simulink model "Model_R2021b"  (R2022b)
settings: Solver=VariableStepAuto  StartTime=0.0  StopTime=10  FixedStep=1e-5  RelTol=1e-3
InitFcn:
  | ModelParameters
values from neighbouring files (symbols this model uses):
  K = lqr(sys, Q, R)    [ModelParameters.m]
  U_ss = [m*g; 0; 0; 0]    [ModelParameters.m]
  X_init = [1.,1.,1.,  0,0,0,  0,0,psi_0, 0,0,0]    [ModelParameters.m]
  X_ref = [0,0,0, 0,0,0, 0,0,psi_t, 0,0,0]    [ModelParameters.m]
settings Model: Creator=samuel  LastModifiedBy=sebas
settings SolverCC: ZeroCrossControl=DisableAll  AlgebraicLoopSolver=TrustRegion
settings DebuggingCC: UnconnectedInputMsg=warning  UnconnectedOutputMsg=warning  UnconnectedLineMsg=warning  UnderSpecifiedDimensionMsg=warning  ArithmeticOperatorsInVariantConditions=warning
settings ModelReferenceCC: EnableRefExpFcnMdlSchedulingChecks=on
settings SFSimCC: CustomCodeUndefinedFunction=UseInterfaceOnly
settings RTWCC: DLArmComputeVersion=19.05

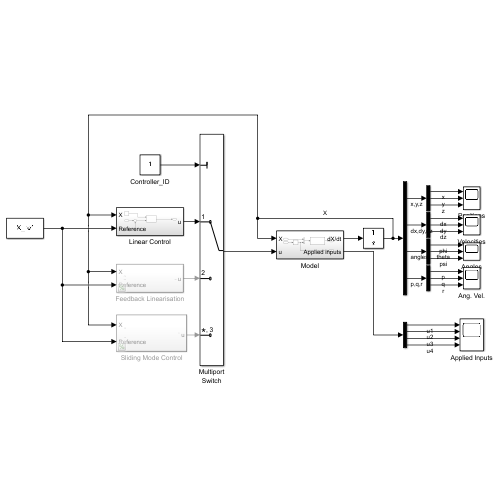
[thumbnail: Simulink's stored preview of the top-level diagram]
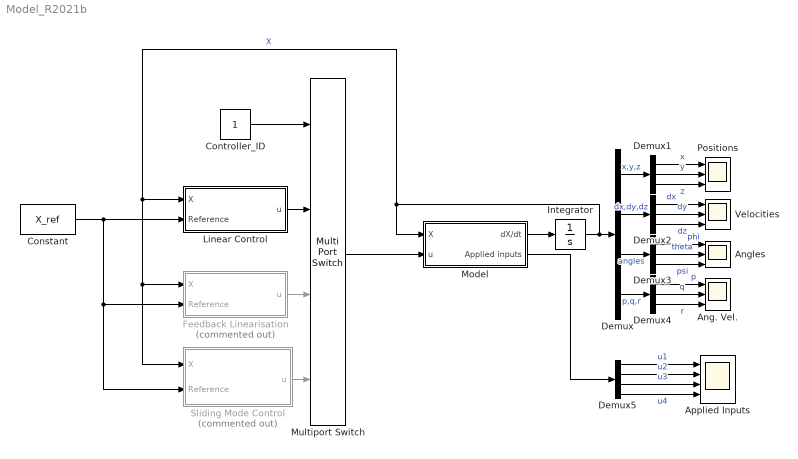
== system Model_R2021b ==
  Ang. Vel. : Scope  NumInputPorts=3
  Angles : Scope  NumInputPorts=3
  "Applied Inputs " : Scope  NumInputPorts=4
  Constant : Constant  Value=X_ref
  Controller_ID : Constant
  Demux : Demux  Outputs=[3,3,3,3]
  Demux{1..4} (4 alike) : Demux  Outputs=3
  Demux5 : Demux
  Feedback Linearisation : Subsystem  Commented=on
  Integrator : Integrator  InitialCondition=X_init
  Linear Control : Subsystem
  Model : Subsystem
  Multiport Switch : MultiPortSwitch  DataPortOrder=Specify indices  SaturateOnIntegerOverflow=off  InputSameDT=off
  Positions : Scope  NumInputPorts=3
  Sliding Mode Control : Subsystem  Commented=on
  Velocities : Scope  NumInputPorts=3
  wires:
  Model/1(dX/dt) -> Integrator/1
  Integrator/1 -> Demux/1, Sliding Mode Control/1(X), Feedback Linearisation/1(X), Linear Control/1(X), Model/1(X)  "X"
  Constant/1 -> Feedback Linearisation/2(Reference), Sliding Mode Control/2(Reference), Linear Control/2(Reference)
  Multiport Switch/1 -> Model/2(u)
  Controller_ID/1 -> Multiport Switch/1
  Feedback Linearisation/1(u) -> Multiport Switch/3
  Linear Control/1(u) -> Multiport Switch/2
  Sliding Mode Control/1(u) -> Multiport Switch/4
  Demux/1 -> Demux1/1  "x,y,z"
  Demux1/1 -> Positions/1  "x"
  Demux1/2 -> Positions/2  "y"
  Demux1/3 -> Positions/3  "z"
  Demux2/2 -> Velocities/2  "dy"
  Demux2/1 -> Velocities/1  "dx"
  Demux2/3 -> Velocities/3  "dz"
  Demux/2 -> Demux2/1  "dx,dy,dz"
  Demux3/1 -> Angles/1  "phi"
  Demux3/3 -> Angles/3  "psi"
  Demux/3 -> Demux3/1  "angles"
  Demux3/2 -> Angles/2  "theta"
  Demux4/2 -> Ang. Vel./2  "q"
  Demux4/1 -> Ang. Vel./1  "p"
  Demux4/3 -> Ang. Vel./3  "r"
  Demux/4 -> Demux4/1  "p,q,r"
  Model/2(Applied inputs) -> Demux5/1
  Demux5/1 -> "Applied Inputs "/1  "u1"
  Demux5/2 -> "Applied Inputs "/2  "u2"
  Demux5/3 -> "Applied Inputs "/3  "u3"
  Demux5/4 -> "Applied Inputs "/4  "u4"

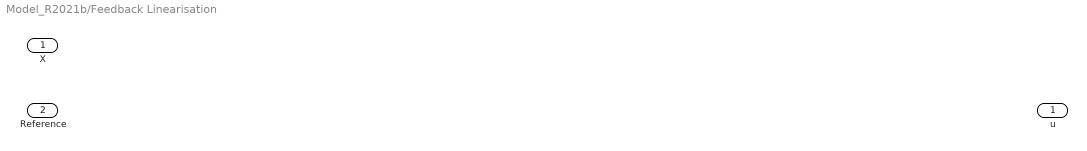
== system Model_R2021b/Feedback Linearisation ==
  X : Inport
  Reference : Inport  Port=2
  u : Outport

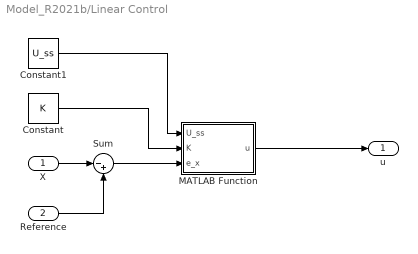
== system Model_R2021b/Linear Control ==
  X : Inport
  Reference : Inport  Port=2
  Constant : Constant  Value=K
  Constant1 : Constant  Value=U_ss
  MATLAB Function : MATLAB Function  TreatAsAtomicUnit=on
  Sum : Sum  Inputs=|-+
  u : Outport
  wires:
  MATLAB Function/1(u) -> u/1
  Constant/1 -> MATLAB Function/2(K)
  X/1 -> Sum/1
  Reference/1 -> Sum/2
  Sum/1 -> MATLAB Function/3(e_x)
  Constant1/1 -> MATLAB Function/1(U_ss)

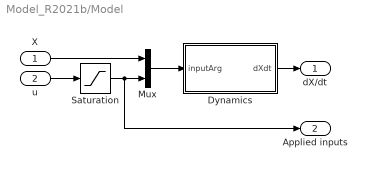
== system Model_R2021b/Model ==
  X : Inport
  u : Inport  Port=2
  Dynamics : MATLAB Function  TreatAsAtomicUnit=on
  Mux : Mux  Inputs=2
  Saturation : Saturate  UpperLimit=10  LowerLimit=-10
  dX/dt : Outport
  Applied inputs : Outport  Port=2
  wires:
  X/1 -> Mux/1
  u/1 -> Saturation/1
  Dynamics/1(dXdt) -> dX/dt/1
  Mux/1 -> Dynamics/1(inputArg)
  Saturation/1 -> Applied inputs/1, Mux/2

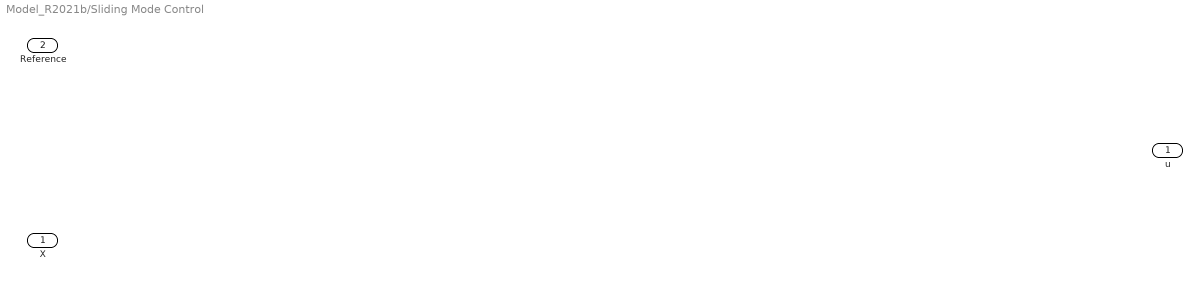
== system Model_R2021b/Sliding Mode Control ==
  X : Inport
  Reference : Inport  Port=2
  u : Outport  VectorParamsAs1DForOutWhenUnconnected=off

== matlab function Model_R2021b/Model/Dynamics ==
  data: inputArg input; dXdt output
function dXdt  = nlmodel(inputArg)
%NLMODEL Compute full state derivative
%   Using non-linear model

%% Parse input

nStates = 12;
nInputs = 4;
% assert(min(size(inputArg) == [1 (nStates + nInputs)]));
X = inputArg(1:nStates);
u = inputArg(nStates + 1:nStates + nInputs);
dXdt = zeros(nStates, 1);

%[x y z dx dy dz theta phi psi p q r] = X;
x       = X(1);
y       = X(2);
z       = X(3);
dx      = X(4);
dy      = X(5);
dz      = X(6);
phi     = X(7);
theta   = X(8);
psi     = X(9);
p       = X(10);
q       = X(11);
r       = X(12);

%% Model parameters

m  = 28e-3;
Ix = 16.57e-6;
Iy = 29.51e-6;
Iz = 29.26e-6;
% 
% m  = 0.65;
% Ix = 7.5e-3;
% Iy = 7.5e-3;
% Iz = 1.3e-2;

Kx = 0.01;
Ky = 0.01;
Kz = 0.01;
Kp = 1e-5;
Kq = 1e-5;
Kr = 1e-5 ;
g  = 9.8;


%% Equations of motion

% 1st derivatives of the position
dXdt(1:3) = X(4:6);

% Eq. 3
dXdt(4) = (1/m) * ((cos(phi)*sin(theta)*cos(psi) + sin(phi)*sin(psi))*u(1) - Kx*dx);
dXdt(5) = (1/m) * ((cos(phi)*sin(theta)*sin(psi) - sin(phi)*cos(psi))*u(1) - Ky*dy);
dXdt(6) = (1/m) * (cos(phi)*cos(theta)*u(1) - m*g - Kz*dz);

% Eq. 1
dXdt(7) = p + q*sin(phi)*tan(theta) +  r*cos(phi)*tan(theta);
dXdt(8) = q*cos(phi) - r*sin(phi);
dXdt(9) = q*sin(phi)/cos(theta) + r*cos(phi)/cos(theta);
         
% Eq. 4
dXdt(10) = (1/Ix)*((Iy-Iz)*q*r + u(2) - Kp*p);
dXdt(11) = (1/Iy)*((Iz-Ix)*p*r + u(3) - Kq*q);
dXdt(12) = (1/Iz)*((Ix-Iy)*p*q + u(4) - Kr*r);

%% Check output dimensions

assert(min(size(dXdt) == [nStates, 1]));
end

== matlab function Model_R2021b/Linear Control/MATLAB Function ==
  data: U_ss input; K input; e_x input; u output
function u = fcn(U_ss, K, e_x)
u = U_ss + K * e_x;
